simulink model "SRSSwSet"  (R2018b)
settings: Solver=FixedStepDiscrete  StartTime=0.0  StopTime=10.0  FixedStep=0.01  RelTol=1e-3
undefined symbols (not defined in the file or in its folder): arg, EEModeList_Set, h1
settings Model: Creator=su3dcu  LastModifiedBy=su3dcu
settings DataIOCC: SaveFormat=StructureWithTime
settings OptimizationCC: DefaultParameterBehavior=Inlined  EnhancedBackFolding=on  PassReuseOutputArgsAs=Individual arguments  ZeroExternalMemoryAtStartup=off  ZeroInternalMemoryAtStartup=off  OptimizeBlockOrder=speed  DifferentSizesBufferReuse=on  OptimizationCustomize=off
settings DebuggingCC: ParameterTunabilityLossMsg=error
settings ModelReferenceCC: ModelReferenceNumInstancesAllowed=Single
settings SFSimCC: MATLABDynamicMemAlloc=off
settings RTWCC: SystemTargetFile=autosar.tlc  GenCodeOnly=on  TemplateMakefile=ert_default_tmf  Description=AUTOSAR  GenerateReport=on  IncludeHyperlinkInReport=on  LaunchReport=on  GenerateTraceInfo=on  GenerateTraceReport=on  GenerateTraceReportSl=on  GenerateTraceReportSf=on  GenerateTraceReportEml=on
settings CodeAppCC: ForceParamTrailComments=on  IgnoreCustomStorageClasses=off  OperatorAnnotations=on  SimulinkDataObjDesc=on  SFDataObjDesc=on  InsertBlockDesc=on
settings STFCustomTargetCC: TargetLangStandard=C99 (ISO)  MultiwordLength=256  ParMdlRefBuildCompliant=on  CompOptLevelCompliant=on  IncludeMdlTerminateFcn=off  CombineOutputUpdateFcns=on  SuppressErrorStatus=on  ERTCustomFileBanners=on  SupportNonFinite=off  SupportComplex=off  SupportContinuousTime=off  SupportNonInlinedSFcns=off  RemoveResetFunc=on  MATLABClassNameForMDSCustomization=Simulink.SoftwareTarget.ERTCustomization  AutosarCompliant=on  UseToolchainInfoCompliant=on  LookupTableObjectStructAxisOrder=2,1,3,4,...  LUTObjectStructOrderEvenSpacing=Size,Table,Breakpoints  SystemTargetFile=autosar.tlc
settings ERTTargetCC: TargetLangStandard=C99 (ISO)  ConcurrentExecutionCompliant=off  IncludeMdlTerminateFcn=off  SuppressErrorStatus=on  SupportNonFinite=off  SupportComplex=off  ModelStepFunctionPrototypeControlCompliant=off  CPPClassGenCompliant=off  AutosarCompliant=on  LookupTableObjectStructAxisOrder=2,1,3,4,...  LUTObjectStructOrderEvenSpacing=Size,Table,Breakpoints  InlinedParameterPlacement=NonHierarchical  ERTCustomFileTemplate=example_file_process.tlc  ERTFilePackagingFormat=Compact

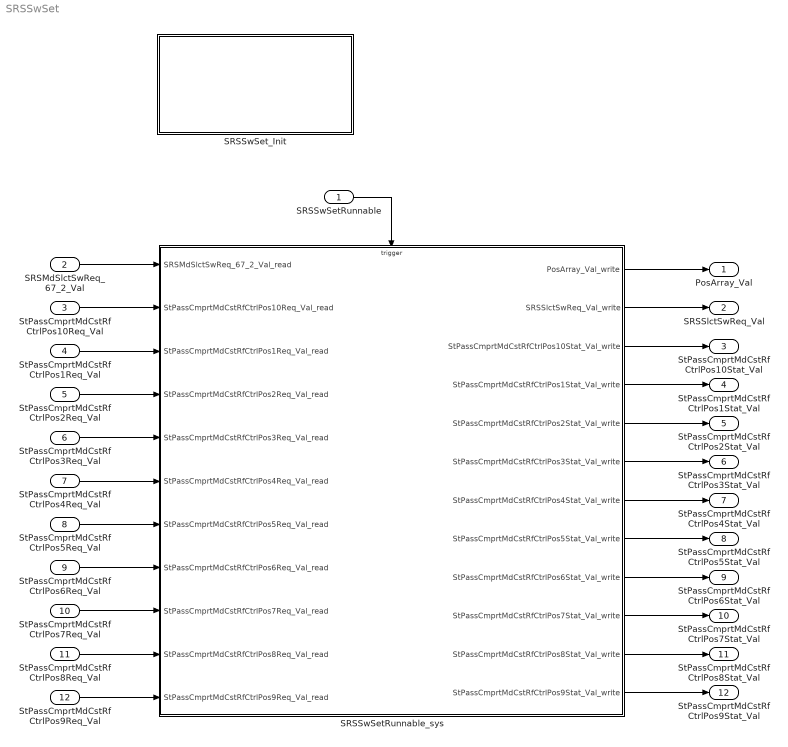
== system SRSSwSet ==
  SRSSwSetRunnable : Inport  SampleTime=0.01  OutputFunctionCall=on
  SRSMdSlctSwReq_67_2_Val : Inport  Port=2  OutDataTypeStr=Enum: SRSSlctSwStat1  PortDimensions=1
  StPassCmprtMdCstRfCtrlPos10Req_Val : Inport  Port=3  OutDataTypeStr=Enum: RfCtrlPosReq  PortDimensions=1
  StPassCmprtMdCstRfCtrlPos1Req_Val : Inport  Port=4  OutDataTypeStr=Enum: RfCtrlPosReq  PortDimensions=1
  StPassCmprtMdCstRfCtrlPos2Req_Val : Inport  Port=5  OutDataTypeStr=Enum: RfCtrlPosReq  PortDimensions=1
  StPassCmprtMdCstRfCtrlPos3Req_Val : Inport  Port=6  OutDataTypeStr=Enum: RfCtrlPosReq  PortDimensions=1
  StPassCmprtMdCstRfCtrlPos4Req_Val : Inport  Port=7  OutDataTypeStr=Enum: RfCtrlPosReq  PortDimensions=1
  StPassCmprtMdCstRfCtrlPos5Req_Val : Inport  Port=8  OutDataTypeStr=Enum: RfCtrlPosReq  PortDimensions=1
  StPassCmprtMdCstRfCtrlPos6Req_Val : Inport  Port=9  OutDataTypeStr=Enum: RfCtrlPosReq  PortDimensions=1
  StPassCmprtMdCstRfCtrlPos7Req_Val : Inport  Port=10  OutDataTypeStr=Enum: RfCtrlPosReq  PortDimensions=1
  StPassCmprtMdCstRfCtrlPos8Req_Val : Inport  Port=11  OutDataTypeStr=Enum: RfCtrlPosReq  PortDimensions=1
  StPassCmprtMdCstRfCtrlPos9Req_Val : Inport  Port=12  OutDataTypeStr=Enum: RfCtrlPosReq  PortDimensions=1
  SRSSwSetRunnable_sys : Subsystem
  SRSSwSet_Init : Subsystem
  PosArray_Val : Outport  OutDataTypeStr=uint8  PortDimensions=11
  SRSSlctSwReq_Val : Outport  Port=2  OutDataTypeStr=Enum: SRSMode1  PortDimensions=1
  StPassCmprtMdCstRfCtrlPos10Stat_Val : Outport  Port=3  OutDataTypeStr=Enum: RfCtrlPosStat  PortDimensions=1
  StPassCmprtMdCstRfCtrlPos1Stat_Val : Outport  Port=4  OutDataTypeStr=Enum: RfCtrlPosStat  PortDimensions=1
  StPassCmprtMdCstRfCtrlPos2Stat_Val : Outport  Port=5  OutDataTypeStr=Enum: RfCtrlPosStat  PortDimensions=1
  StPassCmprtMdCstRfCtrlPos3Stat_Val : Outport  Port=6  OutDataTypeStr=Enum: RfCtrlPosStat  PortDimensions=1
  StPassCmprtMdCstRfCtrlPos4Stat_Val : Outport  Port=7  OutDataTypeStr=Enum: RfCtrlPosStat  PortDimensions=1
  StPassCmprtMdCstRfCtrlPos5Stat_Val : Outport  Port=8  OutDataTypeStr=Enum: RfCtrlPosStat  PortDimensions=1
  StPassCmprtMdCstRfCtrlPos6Stat_Val : Outport  Port=9  OutDataTypeStr=Enum: RfCtrlPosStat  PortDimensions=1
  StPassCmprtMdCstRfCtrlPos7Stat_Val : Outport  Port=10  OutDataTypeStr=Enum: RfCtrlPosStat  PortDimensions=1
  StPassCmprtMdCstRfCtrlPos8Stat_Val : Outport  Port=11  OutDataTypeStr=Enum: RfCtrlPosStat  PortDimensions=1
  StPassCmprtMdCstRfCtrlPos9Stat_Val : Outport  Port=12  OutDataTypeStr=Enum: RfCtrlPosStat  PortDimensions=1
  wires:
  SRSMdSlctSwReq_67_2_Val/1 -> SRSSwSetRunnable_sys/1(SRSMdSlctSwReq_67_2_Val_read)
  StPassCmprtMdCstRfCtrlPos10Req_Val/1 -> SRSSwSetRunnable_sys/2(StPassCmprtMdCstRfCtrlPos10Req_Val_read)
  StPassCmprtMdCstRfCtrlPos1Req_Val/1 -> SRSSwSetRunnable_sys/3(StPassCmprtMdCstRfCtrlPos1Req_Val_read)
  StPassCmprtMdCstRfCtrlPos2Req_Val/1 -> SRSSwSetRunnable_sys/4(StPassCmprtMdCstRfCtrlPos2Req_Val_read)
  StPassCmprtMdCstRfCtrlPos3Req_Val/1 -> SRSSwSetRunnable_sys/5(StPassCmprtMdCstRfCtrlPos3Req_Val_read)
  StPassCmprtMdCstRfCtrlPos4Req_Val/1 -> SRSSwSetRunnable_sys/6(StPassCmprtMdCstRfCtrlPos4Req_Val_read)
  StPassCmprtMdCstRfCtrlPos5Req_Val/1 -> SRSSwSetRunnable_sys/7(StPassCmprtMdCstRfCtrlPos5Req_Val_read)
  StPassCmprtMdCstRfCtrlPos6Req_Val/1 -> SRSSwSetRunnable_sys/8(StPassCmprtMdCstRfCtrlPos6Req_Val_read)
  StPassCmprtMdCstRfCtrlPos7Req_Val/1 -> SRSSwSetRunnable_sys/9(StPassCmprtMdCstRfCtrlPos7Req_Val_read)
  StPassCmprtMdCstRfCtrlPos8Req_Val/1 -> SRSSwSetRunnable_sys/10(StPassCmprtMdCstRfCtrlPos8Req_Val_read)
  StPassCmprtMdCstRfCtrlPos9Req_Val/1 -> SRSSwSetRunnable_sys/11(StPassCmprtMdCstRfCtrlPos9Req_Val_read)
  SRSSwSetRunnable_sys/1(PosArray_Val_write) -> PosArray_Val/1
  SRSSwSetRunnable_sys/2(SRSSlctSwReq_Val_write) -> SRSSlctSwReq_Val/1
  SRSSwSetRunnable_sys/3(StPassCmprtMdCstRfCtrlPos10Stat_Val_write) -> StPassCmprtMdCstRfCtrlPos10Stat_Val/1
  SRSSwSetRunnable_sys/4(StPassCmprtMdCstRfCtrlPos1Stat_Val_write) -> StPassCmprtMdCstRfCtrlPos1Stat_Val/1
  SRSSwSetRunnable_sys/5(StPassCmprtMdCstRfCtrlPos2Stat_Val_write) -> StPassCmprtMdCstRfCtrlPos2Stat_Val/1
  SRSSwSetRunnable_sys/6(StPassCmprtMdCstRfCtrlPos3Stat_Val_write) -> StPassCmprtMdCstRfCtrlPos3Stat_Val/1
  SRSSwSetRunnable_sys/7(StPassCmprtMdCstRfCtrlPos4Stat_Val_write) -> StPassCmprtMdCstRfCtrlPos4Stat_Val/1
  SRSSwSetRunnable_sys/8(StPassCmprtMdCstRfCtrlPos5Stat_Val_write) -> StPassCmprtMdCstRfCtrlPos5Stat_Val/1
  SRSSwSetRunnable_sys/9(StPassCmprtMdCstRfCtrlPos6Stat_Val_write) -> StPassCmprtMdCstRfCtrlPos6Stat_Val/1
  SRSSwSetRunnable_sys/10(StPassCmprtMdCstRfCtrlPos7Stat_Val_write) -> StPassCmprtMdCstRfCtrlPos7Stat_Val/1
  SRSSwSetRunnable_sys/11(StPassCmprtMdCstRfCtrlPos8Stat_Val_write) -> StPassCmprtMdCstRfCtrlPos8Stat_Val/1
  SRSSwSetRunnable_sys/12(StPassCmprtMdCstRfCtrlPos9Stat_Val_write) -> StPassCmprtMdCstRfCtrlPos9Stat_Val/1
  SRSSwSetRunnable/1 -> SRSSwSetRunnable_sys/Trigger

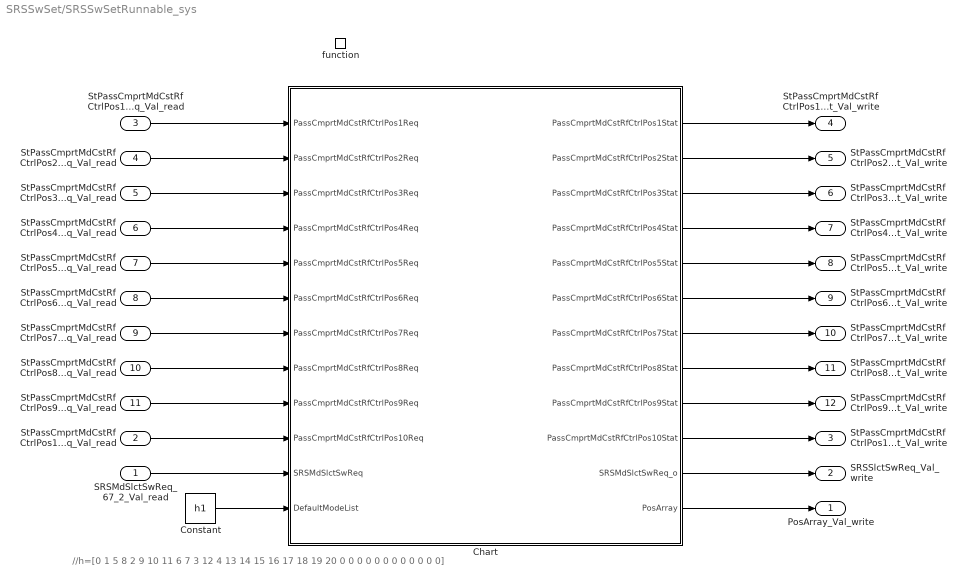
== system SRSSwSet/SRSSwSetRunnable_sys ==
  note: //h=[0 1 5 8 2 9 10 11 6 7 3 12 4 13 14 15 16 17 18 19 20 0 0 0 0 0 0 0 0 0 0 0 0]
  SRSMdSlctSwReq_67_2_Val_read : Inport
  StPassCmprtMdCstRfCtrlPos10Req_Val_read : Inport  Port=2
  StPassCmprtMdCstRfCtrlPos1Req_Val_read : Inport  Port=3
  StPassCmprtMdCstRfCtrlPos2Req_Val_read : Inport  Port=4
  StPassCmprtMdCstRfCtrlPos3Req_Val_read : Inport  Port=5
  StPassCmprtMdCstRfCtrlPos4Req_Val_read : Inport  Port=6
  StPassCmprtMdCstRfCtrlPos5Req_Val_read : Inport  Port=7
  StPassCmprtMdCstRfCtrlPos6Req_Val_read : Inport  Port=8
  StPassCmprtMdCstRfCtrlPos7Req_Val_read : Inport  Port=9
  StPassCmprtMdCstRfCtrlPos8Req_Val_read : Inport  Port=10
  StPassCmprtMdCstRfCtrlPos9Req_Val_read : Inport  Port=11
  function : TriggerPort  TriggerType=function-call  VariantControl=(inherit)  SampleTimeType=periodic  SampleTime=-1
  Chart : Stateflow chart  TreatAsAtomicUnit=on
  Constant : Constant  Value=h1  OutDataTypeStr=uint8
  PosArray_Val_write : Outport
  SRSSlctSwReq_Val_write : Outport  Port=2
  StPassCmprtMdCstRfCtrlPos10Stat_Val_write : Outport  Port=3
  StPassCmprtMdCstRfCtrlPos1Stat_Val_write : Outport  Port=4
  StPassCmprtMdCstRfCtrlPos2Stat_Val_write : Outport  Port=5
  StPassCmprtMdCstRfCtrlPos3Stat_Val_write : Outport  Port=6
  StPassCmprtMdCstRfCtrlPos4Stat_Val_write : Outport  Port=7
  StPassCmprtMdCstRfCtrlPos5Stat_Val_write : Outport  Port=8
  StPassCmprtMdCstRfCtrlPos6Stat_Val_write : Outport  Port=9
  StPassCmprtMdCstRfCtrlPos7Stat_Val_write : Outport  Port=10
  StPassCmprtMdCstRfCtrlPos8Stat_Val_write : Outport  Port=11
  StPassCmprtMdCstRfCtrlPos9Stat_Val_write : Outport  Port=12
  wires:
  Chart/1(PassCmprtMdCstRfCtrlPos1Stat) -> StPassCmprtMdCstRfCtrlPos1Stat_Val_write/1
  Chart/2(PassCmprtMdCstRfCtrlPos2Stat) -> StPassCmprtMdCstRfCtrlPos2Stat_Val_write/1
  Chart/3(PassCmprtMdCstRfCtrlPos3Stat) -> StPassCmprtMdCstRfCtrlPos3Stat_Val_write/1
  Chart/4(PassCmprtMdCstRfCtrlPos4Stat) -> StPassCmprtMdCstRfCtrlPos4Stat_Val_write/1
  Chart/5(PassCmprtMdCstRfCtrlPos5Stat) -> StPassCmprtMdCstRfCtrlPos5Stat_Val_write/1
  Chart/6(PassCmprtMdCstRfCtrlPos6Stat) -> StPassCmprtMdCstRfCtrlPos6Stat_Val_write/1
  Chart/7(PassCmprtMdCstRfCtrlPos7Stat) -> StPassCmprtMdCstRfCtrlPos7Stat_Val_write/1
  Chart/8(PassCmprtMdCstRfCtrlPos8Stat) -> StPassCmprtMdCstRfCtrlPos8Stat_Val_write/1
  Chart/9(PassCmprtMdCstRfCtrlPos9Stat) -> StPassCmprtMdCstRfCtrlPos9Stat_Val_write/1
  Chart/10(PassCmprtMdCstRfCtrlPos10Stat) -> StPassCmprtMdCstRfCtrlPos10Stat_Val_write/1
  Chart/11(SRSMdSlctSwReq_o) -> SRSSlctSwReq_Val_write/1
  Chart/12(PosArray) -> PosArray_Val_write/1
  StPassCmprtMdCstRfCtrlPos1Req_Val_read/1 -> Chart/1(PassCmprtMdCstRfCtrlPos1Req)
  StPassCmprtMdCstRfCtrlPos2Req_Val_read/1 -> Chart/2(PassCmprtMdCstRfCtrlPos2Req)
  StPassCmprtMdCstRfCtrlPos3Req_Val_read/1 -> Chart/3(PassCmprtMdCstRfCtrlPos3Req)
  StPassCmprtMdCstRfCtrlPos4Req_Val_read/1 -> Chart/4(PassCmprtMdCstRfCtrlPos4Req)
  StPassCmprtMdCstRfCtrlPos5Req_Val_read/1 -> Chart/5(PassCmprtMdCstRfCtrlPos5Req)
  StPassCmprtMdCstRfCtrlPos6Req_Val_read/1 -> Chart/6(PassCmprtMdCstRfCtrlPos6Req)
  StPassCmprtMdCstRfCtrlPos7Req_Val_read/1 -> Chart/7(PassCmprtMdCstRfCtrlPos7Req)
  StPassCmprtMdCstRfCtrlPos8Req_Val_read/1 -> Chart/8(PassCmprtMdCstRfCtrlPos8Req)
  StPassCmprtMdCstRfCtrlPos9Req_Val_read/1 -> Chart/9(PassCmprtMdCstRfCtrlPos9Req)
  StPassCmprtMdCstRfCtrlPos10Req_Val_read/1 -> Chart/10(PassCmprtMdCstRfCtrlPos10Req)
  SRSMdSlctSwReq_67_2_Val_read/1 -> Chart/11(SRSMdSlctSwReq)
  Constant/1 -> Chart/12(DefaultModeList)

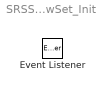
== system SRSSwSet/SRSSwSet_Init ==
  Event Listener : EventListener  EventName=reset

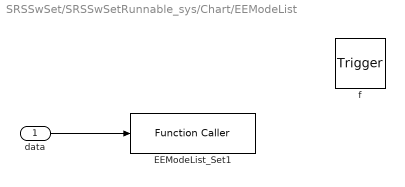
== system SRSSwSet/SRSSwSetRunnable_sys/Chart/EEModeList ==
  data : Inport
  f : TriggerPort  TriggerType=function-call  VariantControl=(inherit)
      settings: CopyFcn=Stateflow.SLINSF.SimulinkMan.removeBlockPreDeleteFcn  PreDeleteFcn=Stateflow.SLINSF.SimulinkMan.unsafePredeleteFcn
  EEModeList_Set1 : FunctionCaller  FunctionPrototype=EEModeList_Set(arg)  InputArgumentSpecifications=uint8([1;1;1;1;1;1;1;1;1;1;1])
  wires:
  data/1 -> EEModeList_Set1/1

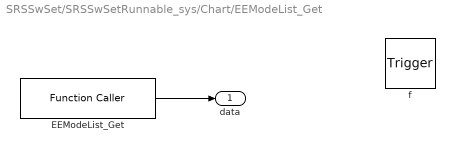
== system SRSSwSet/SRSSwSetRunnable_sys/Chart/EEModeList_Get ==
  f : TriggerPort  TriggerType=function-call  VariantControl=(inherit)
      settings: CopyFcn=Stateflow.SLINSF.SimulinkMan.removeBlockPreDeleteFcn  PreDeleteFcn=Stateflow.SLINSF.SimulinkMan.unsafePredeleteFcn
  EEModeList_Get : FunctionCaller  FunctionPrototype=arg = EEModeList_Get()  OutputArgumentSpecifications=uint8([1;1;1;1;1;1;1;1;1;1;1])
  data : Outport
  wires:
  EEModeList_Get/1 -> data/1

== stateflow chart SRSSwSet/SRSSwSetRunnable_sys/Chart ==
  state Init
    en:
    PosArray = EEModeList_Get();
    PosArray[0] = 0;
    PassCmprtMdCstRfCtrlPos1Req_last = PosArray[1];
    PassCmprtMdCstRfCtrlPos2Req_last = PosArray[2];
    PassCmprtMdCstRfCtrlPos3Req_last = PosArray[3];
    PassCmprtMdCstRfCtrlPos4Req_last = PosArray[4];
    PassCmprtMdCstRfCtrlPos5Req_last = PosArray[5];
    PassCmprtMdCstRfCtrlPos6Req_last = PosArray[6];
    PassCmprtMdCstRfCtrlPos7Req_last = PosArray[7];
    PassCmprtMdCstRfCtrlPos8Req_last = PosArray[8];
    PassCmprtMdCstRfCtrlPos9Req_last = PosArray[9];
    PassCmprtMdCstRfCtrlPos10Req_last = PosArray[10];
  state SetPosReq [function]
    (default) -> (junction 73)
    (junction 75) -> (junction 263) [order 1] : [PassCmprtMdCstRfCtrlPos1Req == RfCtrlPosReq.NoMode]
    (junction 73) -> (junction 75) [order 1] : [(PassCmprtMdCstRfCtrlPos1Req ~= PassCmprtMdCstRfCtrlPos1Req_last) && (PassCmprtMdCstRfCtrlPos1Req != RfCtrlPosReq.NoAction)]
    (junction 75) -> (junction 260) [order 2] : {PosArray[1] = uint8(PassCmprtMdCstRfCtrlPos1Req);}
    (junction 263) -> (junction 262) : {PosArray[1] = uint8(0);}
    (junction 73) -> (junction 332) [order 2]
    (junction 262) -> (junction 260)
    (junction 260) -> (junction 72) : {PassCmprtMdCstRfCtrlPos1Req_last = PassCmprtMdCstRfCtrlPos1Req;
        | EEModeList(PosArray);}
    (junction 72) -> (junction 332)
    (junction 332) -> (junction 79)
    (junction 77) -> (junction 268) [order 1] : [PassCmprtMdCstRfCtrlPos2Req == RfCtrlPosReq.NoMode]
    (junction 79) -> (junction 77) [order 1] : [(PassCmprtMdCstRfCtrlPos2Req ~= PassCmprtMdCstRfCtrlPos2Req_last) && (PassCmprtMdCstRfCtrlPos2Req != RfCtrlPosReq.NoAction)]
    (junction 77) -> (junction 272) [order 2] : {PosArray[2] = uint8(PassCmprtMdCstRfCtrlPos2Req);}
    (junction 268) -> (junction 270) : {PosArray[2] = uint8(0);}
    (junction 79) -> (junction 335) [order 2]
    (junction 270) -> (junction 272)
    (junction 272) -> (junction 81) : {PassCmprtMdCstRfCtrlPos2Req_last = PassCmprtMdCstRfCtrlPos2Req;
        | EEModeList(PosArray);}
    (junction 81) -> (junction 335)
    (junction 335) -> (junction 89)
    (junction 89) -> (junction 83) [order 1] : [(PassCmprtMdCstRfCtrlPos3Req ~= PassCmprtMdCstRfCtrlPos3Req_last) && (PassCmprtMdCstRfCtrlPos3Req != RfCtrlPosReq.NoAction)]
    (junction 83) -> (junction 275) [order 1] : [PassCmprtMdCstRfCtrlPos3Req == RfCtrlPosReq.NoMode]
    (junction 89) -> (junction 338) [order 2]
    (junction 83) -> (junction 279) [order 2] : {PosArray[3] = uint8(PassCmprtMdCstRfCtrlPos3Req);}
    (junction 275) -> (junction 276) : {PosArray[3] = uint8(0);}
    (junction 276) -> (junction 279)
    (junction 279) -> (junction 87) : {PassCmprtMdCstRfCtrlPos3Req_last = PassCmprtMdCstRfCtrlPos3Req;
        | EEModeList(PosArray);}
    (junction 87) -> (junction 338)
    (junction 338) -> (junction 80)
    (junction 92) -> (junction 282) [order 1] : [PassCmprtMdCstRfCtrlPos4Req == RfCtrlPosReq.NoMode]
    (junction 80) -> (junction 92) [order 1] : [(PassCmprtMdCstRfCtrlPos4Req ~= PassCmprtMdCstRfCtrlPos4Req_last) && (PassCmprtMdCstRfCtrlPos4Req != RfCtrlPosReq.NoAction)]
    (junction 282) -> (junction 283) : {PosArray[4] = uint8(0);}
    (junction 92) -> (junction 284) [order 2] : {PosArray[4] = uint8(PassCmprtMdCstRfCtrlPos4Req);}
    (junction 80) -> (junction 341) [order 2]
    (junction 283) -> (junction 284)
    (junction 284) -> (junction 91) : {PassCmprtMdCstRfCtrlPos4Req_last = PassCmprtMdCstRfCtrlPos4Req;
        | EEModeList(PosArray);}
    (junction 91) -> (junction 341)
    (junction 341) -> (junction 96)
    (junction 95) -> (junction 289) [order 1] : [PassCmprtMdCstRfCtrlPos5Req == RfCtrlPosReq.NoMode]
    (junction 96) -> (junction 95) [order 1] : [(PassCmprtMdCstRfCtrlPos5Req ~= PassCmprtMdCstRfCtrlPos5Req_last) && (PassCmprtMdCstRfCtrlPos5Req != RfCtrlPosReq.NoAction)]
    (junction 95) -> (junction 291) [order 2] : {PosArray[5] = uint8(PassCmprtMdCstRfCtrlPos5Req);}
    (junction 289) -> (junction 290) : {PosArray[5] = uint8(0);}
    (junction 96) -> (junction 344) [order 2]
    (junction 290) -> (junction 291)
    (junction 291) -> (junction 98) : {PassCmprtMdCstRfCtrlPos5Req_last = PassCmprtMdCstRfCtrlPos5Req;
        | EEModeList(PosArray);}
    (junction 98) -> (junction 344)
    (junction 344) -> (junction 100)
    (junction 102) -> (junction 296) [order 1] : [PassCmprtMdCstRfCtrlPos6Req == RfCtrlPosReq.NoMode]
    (junction 100) -> (junction 102) [order 1] : [(PassCmprtMdCstRfCtrlPos6Req ~= PassCmprtMdCstRfCtrlPos6Req_last) && (PassCmprtMdCstRfCtrlPos6Req != RfCtrlPosReq.NoAction)]
    (junction 102) -> (junction 300) [order 2] : {PosArray[6] = uint8(PassCmprtMdCstRfCtrlPos6Req);}
    (junction 296) -> (junction 297) : {PosArray[6] = uint8(0);}
    (junction 100) -> (junction 347) [order 2]
    (junction 297) -> (junction 300)
    (junction 300) -> (junction 104) : {PassCmprtMdCstRfCtrlPos6Req_last = PassCmprtMdCstRfCtrlPos6Req;
        | EEModeList(PosArray);}
    (junction 104) -> (junction 347)
    (junction 347) -> (junction 106)
    (junction 106) -> (junction 108) [order 1] : [(PassCmprtMdCstRfCtrlPos7Req ~= PassCmprtMdCstRfCtrlPos7Req_last) && (PassCmprtMdCstRfCtrlPos7Req != RfCtrlPosReq.NoAction)]
    (junction 108) -> (junction 303) [order 1] : [PassCmprtMdCstRfCtrlPos7Req == RfCtrlPosReq.NoMode]
    (junction 106) -> (junction 350) [order 2]
    (junction 108) -> (junction 305) [order 2] : {PosArray[7] = uint8(PassCmprtMdCstRfCtrlPos7Req);}
    (junction 303) -> (junction 304) : {PosArray[7] = uint8(0);}
    (junction 304) -> (junction 305)
    (junction 305) -> (junction 110) : {PassCmprtMdCstRfCtrlPos7Req_last = PassCmprtMdCstRfCtrlPos7Req;
        | EEModeList(PosArray);}
    (junction 110) -> (junction 350)
    (junction 350) -> (junction 112)
    (junction 112) -> (junction 113) [order 1] : [(PassCmprtMdCstRfCtrlPos8Req ~= PassCmprtMdCstRfCtrlPos8Req_last)&& (PassCmprtMdCstRfCtrlPos8Req != RfCtrlPosReq.NoAction)]
    (junction 113) -> (junction 310) [order 1] : [PassCmprtMdCstRfCtrlPos8Req == RfCtrlPosReq.NoMode]
    (junction 112) -> (junction 353) [order 2]
    (junction 113) -> (junction 312) [order 2] : {PosArray[8] = uint8(PassCmprtMdCstRfCtrlPos8Req);}
    (junction 310) -> (junction 311) : {PosArray[8] = uint8(0);}
    (junction 311) -> (junction 312)
    (junction 312) -> (junction 116) : {PassCmprtMdCstRfCtrlPos8Req_last = PassCmprtMdCstRfCtrlPos8Req;
        | EEModeList(PosArray);}
    (junction 116) -> (junction 353)
    (junction 353) -> (junction 118)
    (junction 118) -> (junction 120) [order 1] : [(PassCmprtMdCstRfCtrlPos9Req ~= PassCmprtMdCstRfCtrlPos9Req_last)&& (PassCmprtMdCstRfCtrlPos9Req != RfCtrlPosReq.NoAction)]
    (junction 120) -> (junction 318) [order 1] : [PassCmprtMdCstRfCtrlPos9Req == RfCtrlPosReq.NoMode]
    (junction 118) -> (junction 356) [order 2]
    (junction 120) -> (junction 320) [order 2] : {PosArray[9] = uint8(PassCmprtMdCstRfCtrlPos9Req);}
    (junction 318) -> (junction 319) : {PosArray[9] = uint8(0);}
    (junction 319) -> (junction 320)
    (junction 320) -> (junction 122) : {PassCmprtMdCstRfCtrlPos9Req_last = PassCmprtMdCstRfCtrlPos9Req;
        | EEModeList(PosArray);}
    (junction 122) -> (junction 356)
    (junction 356) -> (junction 124)
    (junction 124) -> (junction 127) [order 1] : [(PassCmprtMdCstRfCtrlPos10Req ~= PassCmprtMdCstRfCtrlPos10Req_last)&& (PassCmprtMdCstRfCtrlPos10Req != RfCtrlPosReq.NoAction)]
    (junction 127) -> (junction 325) [order 1] : [PassCmprtMdCstRfCtrlPos10Req == RfCtrlPosReq.NoMode]
    (junction 124) -> (junction 131) [order 2]
    (junction 127) -> (junction 327) [order 2] : {PosArray[10] = uint8(PassCmprtMdCstRfCtrlPos10Req);}
    (junction 325) -> (junction 326) : {PosArray[10] = uint8(0);}
    (junction 326) -> (junction 327)
    (junction 327) -> (junction 129) : {PassCmprtMdCstRfCtrlPos10Req_last = PassCmprtMdCstRfCtrlPos10Req;
        | EEModeList(PosArray);}
    (junction 129) -> (junction 131)
    (junction 131) -> (junction 143)
  state data = EEModeList_Get [function]
  state EEModeList(data) [function]
  state SlctSwPos [function]
    (default) -> (junction 152)
    (junction 152) -> (junction 154) : {index_i = PosArray[uint8(SRSMdSlctSwReq)]}
    (junction 154) -> (junction 159) : {SRSMdSlctSwReq_o = SRSMode1(DefaultModeList[index_i])}
  state SetPosStat [function]
    (default) -> (junction 164)
    (junction 164) -> (junction 166) [order 1] : [PassCmprtMdCstRfCtrlPos1Req == RfCtrlPosReq.NoMode]
    (junction 166) -> (junction 171) : {PassCmprtMdCstRfCtrlPos1Stat = RfCtrlPosStat.NoModeSet;}
    (junction 164) -> (junction 173) [order 2] : {PassCmprtMdCstRfCtrlPos1Stat =RfCtrlPosStat(PassCmprtMdCstRfCtrlPos1Req_last)}
    (junction 171) -> (junction 173)
    (junction 173) -> (junction 176)
    (junction 176) -> (junction 178) [order 1] : [PassCmprtMdCstRfCtrlPos2Req == RfCtrlPosReq.NoMode]
    (junction 176) -> (junction 182) [order 2] : {PassCmprtMdCstRfCtrlPos2Stat =RfCtrlPosStat(PassCmprtMdCstRfCtrlPos2Req_last)}
    (junction 178) -> (junction 180) : {PassCmprtMdCstRfCtrlPos2Stat = RfCtrlPosStat.NoModeSet;}
    (junction 180) -> (junction 182)
    (junction 182) -> (junction 185)
    (junction 185) -> (junction 187) [order 1] : [PassCmprtMdCstRfCtrlPos3Req == RfCtrlPosReq.NoMode]
    (junction 187) -> (junction 189) : {PassCmprtMdCstRfCtrlPos3Stat = RfCtrlPosStat.NoModeSet;}
    (junction 185) -> (junction 191) [order 2] : {PassCmprtMdCstRfCtrlPos3Stat =RfCtrlPosStat(PassCmprtMdCstRfCtrlPos3Req_last)}
    (junction 189) -> (junction 191)
    (junction 191) -> (junction 194)
    (junction 194) -> (junction 196) [order 1] : [PassCmprtMdCstRfCtrlPos4Req == RfCtrlPosReq.NoMode]
    (junction 196) -> (junction 198) : {PassCmprtMdCstRfCtrlPos4Stat = RfCtrlPosStat.NoModeSet;}
    (junction 194) -> (junction 200) [order 2] : {PassCmprtMdCstRfCtrlPos4Stat =RfCtrlPosStat(PassCmprtMdCstRfCtrlPos4Req_last)}
    (junction 198) -> (junction 200)
    (junction 200) -> (junction 203)
    (junction 203) -> (junction 205) [order 1] : [PassCmprtMdCstRfCtrlPos5Req == RfCtrlPosReq.NoMode]
    (junction 203) -> (junction 209) [order 2] : {PassCmprtMdCstRfCtrlPos5Stat =RfCtrlPosStat(PassCmprtMdCstRfCtrlPos5Req_last)}
    (junction 205) -> (junction 207) : {PassCmprtMdCstRfCtrlPos5Stat = RfCtrlPosStat.NoModeSet;}
    (junction 207) -> (junction 209)
    (junction 209) -> (junction 212)
    (junction 212) -> (junction 214) [order 1] : [PassCmprtMdCstRfCtrlPos6Req == RfCtrlPosReq.NoMode]
    (junction 212) -> (junction 218) [order 2] : {PassCmprtMdCstRfCtrlPos6Stat =RfCtrlPosStat(PassCmprtMdCstRfCtrlPos6Req_last)}
    (junction 214) -> (junction 216) : {PassCmprtMdCstRfCtrlPos6Stat = RfCtrlPosStat.NoModeSet;}
    (junction 216) -> (junction 218)
    (junction 218) -> (junction 221)
    (junction 221) -> (junction 223) [order 1] : [PassCmprtMdCstRfCtrlPos7Req == RfCtrlPosReq.NoMode]
    (junction 221) -> (junction 227) [order 2] : {PassCmprtMdCstRfCtrlPos7Stat =RfCtrlPosStat(PassCmprtMdCstRfCtrlPos7Req_last)}
    (junction 223) -> (junction 225) : {PassCmprtMdCstRfCtrlPos7Stat = RfCtrlPosStat.NoModeSet;}
    (junction 225) -> (junction 227)
    (junction 227) -> (junction 230)
    (junction 230) -> (junction 232) [order 1] : [PassCmprtMdCstRfCtrlPos8Req == RfCtrlPosReq.NoMode]
    (junction 230) -> (junction 234) [order 2] : {PassCmprtMdCstRfCtrlPos8Stat =RfCtrlPosStat(PassCmprtMdCstRfCtrlPos8Req_last)}
    (junction 232) -> (junction 236) : {PassCmprtMdCstRfCtrlPos8Stat = RfCtrlPosStat.NoModeSet;}
    (junction 236) -> (junction 234)
    (junction 234) -> (junction 239)
    (junction 239) -> (junction 241) [order 1] : [PassCmprtMdCstRfCtrlPos9Req == RfCtrlPosReq.NoMode]
    (junction 241) -> (junction 243) : {PassCmprtMdCstRfCtrlPos9Stat = RfCtrlPosStat.NoModeSet;}
    (junction 239) -> (junction 245) [order 2] : {PassCmprtMdCstRfCtrlPos9Stat =RfCtrlPosStat(PassCmprtMdCstRfCtrlPos9Req_last)}
    (junction 243) -> (junction 245)
    (junction 245) -> (junction 248)
    (junction 248) -> (junction 250) [order 1] : [PassCmprtMdCstRfCtrlPos10Req == RfCtrlPosReq.NoMode]
    (junction 248) -> (junction 254) [order 2] : {PassCmprtMdCstRfCtrlPos10Stat =RfCtrlPosStat(PassCmprtMdCstRfCtrlPos10Req_last)}
    (junction 250) -> (junction 252) : {PassCmprtMdCstRfCtrlPos10Stat = RfCtrlPosStat.NoModeSet;}
    (junction 252) -> (junction 254)
    (junction 254) -> (junction 257)
  state SetPosState
    du:
    SetPosReq();
    SetPosStat();
    SlctSwPos();
  (default) -> Init
  Init -> SetPosState
  data: data function_output; data function_input; index_i local uint8; PassCmprtMdCstRfCtrlPos1Req_last local Enum: RfCtrlPosReq size=1; PassCmprtMdCstRfCtrlPos2Req_last local Enum: RfCtrlPosReq size=1; PassCmprtMdCstRfCtrlPos3Req_last local Enum: RfCtrlPosReq size=1; PassCmprtMdCstRfCtrlPos4Req_last local Enum: RfCtrlPosReq size=1; PassCmprtMdCstRfCtrlPos5Req_last local Enum: RfCtrlPosReq size=1; PassCmprtMdCstRfCtrlPos6Req_last local Enum: RfCtrlPosReq size=1; PassCmprtMdCstRfCtrlPos7Req_last local Enum: RfCtrlPosReq size=1; PassCmprtMdCstRfCtrlPos8Req_last local Enum: RfCtrlPosReq size=1; PassCmprtMdCstRfCtrlPos9Req_last local Enum: RfCtrlPosReq size=1; PassCmprtMdCstRfCtrlPos10Req_last local Enum: RfCtrlPosReq size=1; PassCmprtMdCstRfCtrlPos1Stat output Enum: RfCtrlPosStat; PassCmprtMdCstRfCtrlPos2Stat output Enum: RfCtrlPosStat; PassCmprtMdCstRfCtrlPos3Stat output Enum: RfCtrlPosStat; PassCmprtMdCstRfCtrlPos4Stat output Enum: RfCtrlPosStat; PassCmprtMdCstRfCtrlPos5Stat output Enum: RfCtrlPosStat; PassCmprtMdCstRfCtrlPos6Stat output Enum: RfCtrlPosStat; PassCmprtMdCstRfCtrlPos7Stat output Enum: RfCtrlPosStat; PassCmprtMdCstRfCtrlPos8Stat output Enum: RfCtrlPosStat; PassCmprtMdCstRfCtrlPos9Stat output Enum: RfCtrlPosStat; PassCmprtMdCstRfCtrlPos10Stat output Enum: RfCtrlPosStat; PassCmprtMdCstRfCtrlPos1Req input Enum: RfCtrlPosReq; PassCmprtMdCstRfCtrlPos2Req input Enum: RfCtrlPosReq; PassCmprtMdCstRfCtrlPos3Req input Enum: RfCtrlPosReq; PassCmprtMdCstRfCtrlPos4Req input Enum: RfCtrlPosReq; PassCmprtMdCstRfCtrlPos5Req input Enum: RfCtrlPosReq; PassCmprtMdCstRfCtrlPos6Req input Enum: RfCtrlPosReq; PassCmprtMdCstRfCtrlPos7Req input Enum: RfCtrlPosReq; PassCmprtMdCstRfCtrlPos8Req input Enum: RfCtrlPosReq; PassCmprtMdCstRfCtrlPos9Req input Enum: RfCtrlPosReq; PassCmprtMdCstRfCtrlPos10Req input Enum: RfCtrlPosReq; SRSMdSlctSwReq input Enum: SRSSlctSwStat1; SRSMdSlctSwReq_o output Enum: SRSMode1; DefaultModeList input uint8 size=33 =[0,1,5,2,8,9,10,11,6,7,3,12,4,13,14,15,0,0,0,0,0,0,0,0,0,0,0,0,0,0,0,0]; PosArray output uint8 size=11
